simulink model "GFLIB_Limit_BAM_F16"  (Simulink 8.3)
settings: Solver=ode45  StartTime=0.0  StopTime=10.0  RelTol=1e-3
undefined symbols (not defined in the file): f16LowerLim, f16UpperLimit
settings Model: Creator=B17364  LastModifiedBy=B17364
settings OptimizationCC: ExpressionDepthLimit=2147483647
settings DebuggingCC: FcnCallInpInsideContextMsg=UseLocalSettings  StrictBusMsg=Warning

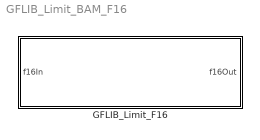
== system GFLIB_Limit_BAM_F16 ==
  GFLIB_Limit_F16 : Subsystem  mask(GFLIB_Limit){f16UpperLimit=f16UpperLimit, f16LowerLim=f16LowerLim}
      mask help: Bit accurate model of the GFLIB_Limit function.
      mask init:
      | pos = get_param(gcb, 'Position');width = pos(3) - pos(1); height = pos(4) - pos(2);tX=width/2;tY=height*0.9;
      mask Display: color('black');port_label('input',1,'f16In');port_label('output',1,'f16Out');color('black');disp('GFLIB_Limit_F16');color('blue');text(tX,tY, 'BAM', 'horizontalAlignment', 'center');

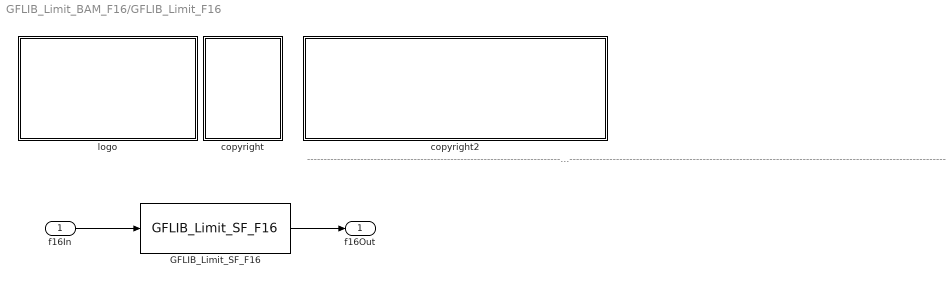
== system GFLIB_Limit_BAM_F16/GFLIB_Limit_F16 ==
  note: ---------------------------------------------------------------------------------------------------------------------------------------------------------------------------------------------------
  f16In : Inport
  GFLIB_Limit_SF_F16 : S-Function  FunctionName=GFLIB_Limit_SF_F16  Parameters=f16UpperLimit,f16LowerLim  EnableBusSupport=off
  copyright : Subsystem
      mask Display:
      | text(10,90,'FILE:');text(10,75,'DESRIPTION:')
      | text(10,60,'COPYRIGHT:')
      | text(10,45,'VERSION:')
      | text(10,30,'DATE:')
      | text(10,15,'AUTHOR:')
  copyright2 : Subsystem
      mask Display:
      | text(10,90,'GFLIB_Limit_BAM_F16.mdl');text(10,75,'Limit function');text(10,60,'Freescale')
      | text(10,45,'0.1');text(10,30,'03-Jul-2011');text(10,15,'');
  logo : Subsystem
      mask Display: image(imread('logo.jpg'))
  f16Out : Outport
  wires:
  f16In/1 -> GFLIB_Limit_SF_F16/1
  GFLIB_Limit_SF_F16/1 -> f16Out/1

== system GFLIB_Limit_BAM_F16/GFLIB_Limit_F16/copyright ==

== system GFLIB_Limit_BAM_F16/GFLIB_Limit_F16/copyright2 ==

== system GFLIB_Limit_BAM_F16/GFLIB_Limit_F16/logo ==
